simulink model "Q3_SIM"  (R2021b)
settings: Solver=VariableStepAuto  StartTime=0.0  StopTime=5  RelTol=1e-3
undefined symbols (not defined in the file): Gd_Bilinear_T1, Gd_Bilinear_T2, Gd_Bilinear_T3, Gd_ZPmatched_T1, Gd_ZPmatched_T2, Gd_ZPmatched_T3, Gd_ZPmatched_T4, gp, Ts
settings Model: Creator=Lenovo  LastModifiedBy=Lenovo

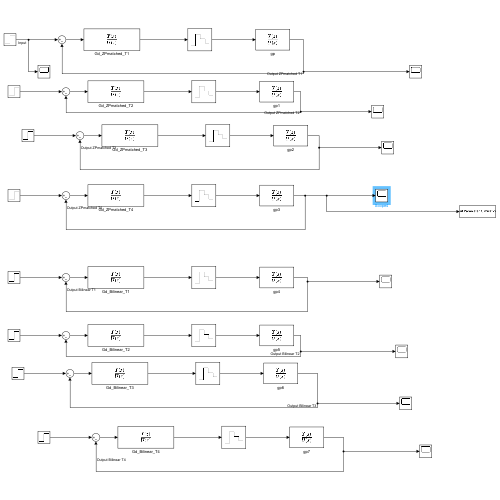
[thumbnail: Simulink's stored preview of the top-level diagram]
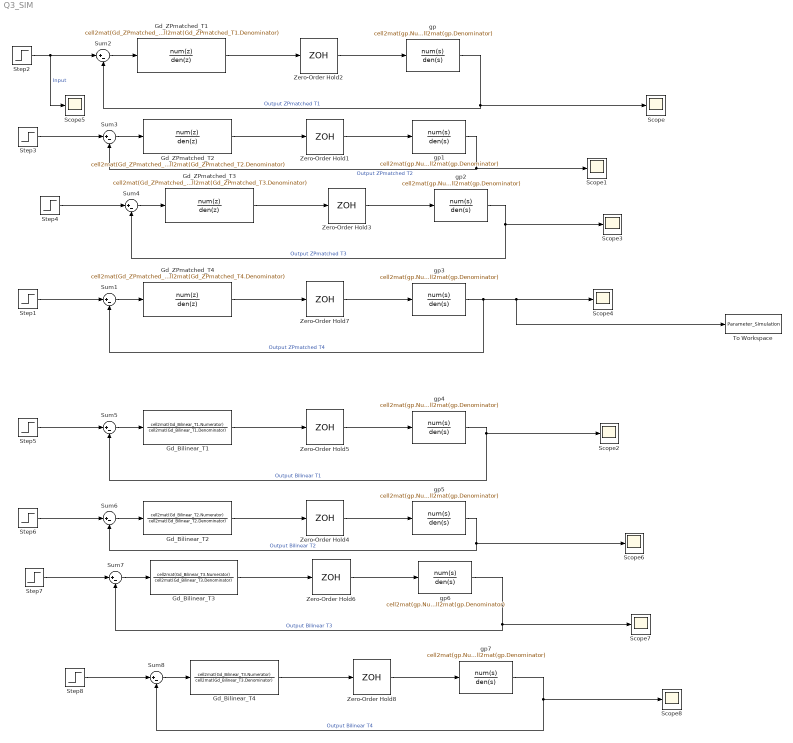
== system Q3_SIM ==
  Gd_Bilinear_T1 : DiscreteTransferFcn  Numerator=cell2mat(Gd_Bilinear_T1.Numerator)  Denominator=cell2mat(Gd_Bilinear_T1.Denominator)  SampleTime=Ts(1)
  Gd_Bilinear_T2 : DiscreteTransferFcn  Numerator=cell2mat(Gd_Bilinear_T2.Numerator)  Denominator=cell2mat(Gd_Bilinear_T2.Denominator)  SampleTime=Ts(2)
  Gd_Bilinear_T3 : DiscreteTransferFcn  Numerator=cell2mat(Gd_Bilinear_T3.Numerator)  Denominator=cell2mat(Gd_Bilinear_T3.Denominator)  SampleTime=Ts(3)
  Gd_Bilinear_T4 : DiscreteTransferFcn  Numerator=cell2mat(Gd_Bilinear_T3.Numerator)  Denominator=cell2mat(Gd_Bilinear_T3.Denominator)  SampleTime=Ts(4)
  Gd_ZPmatched_T1 : DiscreteTransferFcn  Numerator=cell2mat(Gd_ZPmatched_T1.Numerator)  Denominator=cell2mat(Gd_ZPmatched_T1.Denominator)  SampleTime=Ts(1)
  Gd_ZPmatched_T2 : DiscreteTransferFcn  Numerator=cell2mat(Gd_ZPmatched_T2.Numerator)  Denominator=cell2mat(Gd_ZPmatched_T2.Denominator)  SampleTime=Ts(2)
  Gd_ZPmatched_T3 : DiscreteTransferFcn  Numerator=cell2mat(Gd_ZPmatched_T3.Numerator)  Denominator=cell2mat(Gd_ZPmatched_T3.Denominator)  SampleTime=Ts(3)
  Gd_ZPmatched_T4 : DiscreteTransferFcn  Numerator=cell2mat(Gd_ZPmatched_T4.Numerator)  Denominator=cell2mat(Gd_ZPmatched_T4.Denominator)  SampleTime=Ts(4)
  Scope{,1..8} (9 alike) : Scope
  Step{1..8} (8 alike) : Step  Time=0  After=0.0001  SampleTime=0
  Sum{1..8} (8 alike) : Sum  Inputs=|+-
  To Workspace : ToWorkspace  VariableName=Parameter_Simulation  SaveFormat=Timeseries  SampleTime=-1
  Zero-Order Hold1 : ZeroOrderHold  SampleTime=Ts(2)
  Zero-Order Hold2 : ZeroOrderHold  SampleTime=Ts(1)
  Zero-Order Hold3 : ZeroOrderHold  SampleTime=Ts(3)
  Zero-Order Hold4 : ZeroOrderHold  SampleTime=Ts(2)
  Zero-Order Hold5 : ZeroOrderHold  SampleTime=Ts(1)
  Zero-Order Hold6 : ZeroOrderHold  SampleTime=Ts(3)
  Zero-Order Hold7 : ZeroOrderHold  SampleTime=Ts(4)
  Zero-Order Hold8 : ZeroOrderHold  SampleTime=Ts(4)
  gp{,1..7} (8 alike) : TransferFcn  Numerator=cell2mat(gp.Numerator)  Denominator=cell2mat(gp.Denominator)
  wires:
  Step7/1 -> Sum7/1
  Sum2/1 -> Gd_ZPmatched_T1/1
  Gd_ZPmatched_T1/1 -> Zero-Order Hold2/1
  gp/1 -> Scope/1, Sum2/2  "Output ZPmatched T1"
  Zero-Order Hold1/1 -> gp1/1
  Sum3/1 -> Gd_ZPmatched_T2/1
  Gd_ZPmatched_T3/1 -> Zero-Order Hold3/1
  Zero-Order Hold3/1 -> gp2/1
  Step5/1 -> Sum5/1
  Gd_Bilinear_T1/1 -> Zero-Order Hold5/1
  Sum5/1 -> Gd_Bilinear_T1/1
  Sum4/1 -> Gd_ZPmatched_T3/1
  Zero-Order Hold4/1 -> gp5/1
  Gd_ZPmatched_T2/1 -> Zero-Order Hold1/1
  Sum7/1 -> Gd_Bilinear_T3/1
  Step2/1 -> Scope5/1, Sum2/1  "Input"
  Zero-Order Hold2/1 -> gp/1
  Step4/1 -> Sum4/1
  Step6/1 -> Sum6/1
  gp2/1 -> Sum4/2, Scope3/1  "Output ZPmatched T3"
  gp4/1 -> Sum5/2, Scope2/1  "Output Bilinear T1"
  Gd_Bilinear_T2/1 -> Zero-Order Hold4/1
  gp6/1 -> Scope7/1, Sum7/2  "Output Bilinear T3"
  gp1/1 -> Scope1/1, Sum3/2  "Output ZPmatched T2"
  gp5/1 -> Scope6/1, Sum6/2  "Output Bilinear T2"
  Gd_Bilinear_T3/1 -> Zero-Order Hold6/1
  Step3/1 -> Sum3/1
  Zero-Order Hold6/1 -> gp6/1
  Sum6/1 -> Gd_Bilinear_T2/1
  Zero-Order Hold5/1 -> gp4/1
  Step1/1 -> Sum1/1
  gp3/1 -> Sum1/2, To Workspace/1, Scope4/1  "Output ZPmatched T4"
  Sum1/1 -> Gd_ZPmatched_T4/1
  Zero-Order Hold7/1 -> gp3/1
  Gd_ZPmatched_T4/1 -> Zero-Order Hold7/1
  gp7/1 -> Scope8/1, Sum8/2  "Output Bilinear T4"
  Sum8/1 -> Gd_Bilinear_T4/1
  Zero-Order Hold8/1 -> gp7/1
  Step8/1 -> Sum8/1
  Gd_Bilinear_T4/1 -> Zero-Order Hold8/1
